simulink model "Assignment_2_simulink"  (R2025a)
settings: Solver=FixedStepDiscrete  StartTime=0.0  StopTime=inf  FixedStep=0.1  RelTol=1e-3  EnableMultiTasking=on
values from neighbouring files (symbols this model uses):
  Kv = 0.35    [Assignment_2.m]
  Kw = 2    [Assignment_2.m]
  Quaternion_Matrix = [waypoints(:, 1:2) Quaternion_Matrix]    [Assignment_2.m]
  tol = 0.05    [Assignment_2.m]
undefined symbols (not defined in the file or in its folder): twist
libraries: ros2lib x4
settings Model: Creator=arrigon88_msi_u24  LastModifiedBy=diego
settings OptimizationCC: DefaultParameterBehavior=Inlined  EnhancedBackFolding=on  PassReuseOutputArgsAs=Individual arguments  ZeroExternalMemoryAtStartup=off  ZeroInternalMemoryAtStartup=off  MaxStackSize=64  OptimizeBlockOrder=speed  DifferentSizesBufferReuse=on  OptimizationCustomize=off  EfficientTunableParamExpr=on
settings DebuggingCC: ParameterTunabilityLossMsg=error
settings HardwareCC: ProdBitPerLong=64.0  ProdHWDeviceType=Intel->x86-64 (Linux 64)
settings SFSimCC: MATLABDynamicMemAlloc=off
settings RTWCC: SystemTargetFile=ert.tlc  HardwareBoard=Robot Operating System 2 (ROS 2)  TLCOptions="-aInlineSetEventsForThisBaseRateFcn=TLC_FALSE -aSuppressMultiTaskScheduler=TLC_FALSE  -aRateBasedStepFcn=0"  TemplateMakefile=ert_default_tmf  Toolchain=Colcon Tools  TargetLang=C++  Description=Embedded Coder
settings CodeAppCC: ForceParamTrailComments=on  IgnoreCustomStorageClasses=off  OperatorAnnotations=on  SimulinkDataObjDesc=on  SFDataObjDesc=on  InsertBlockDesc=on
settings ERTTargetCC: ExtModeTransport=2.0  ExtModeAutomaticAllocSize=off  RootIOFormat=Structure reference  CodeInterfacePackaging=C++ class

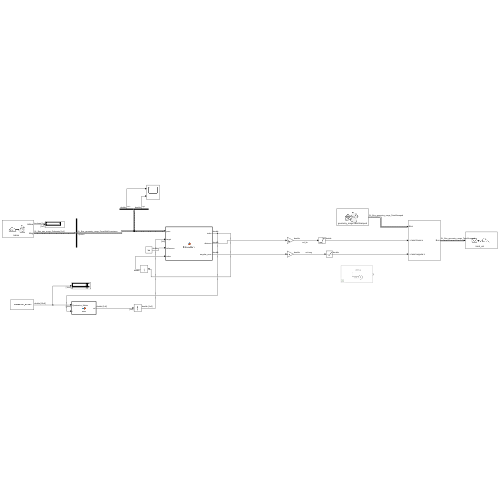
[thumbnail: Simulink's stored preview of the top-level diagram]
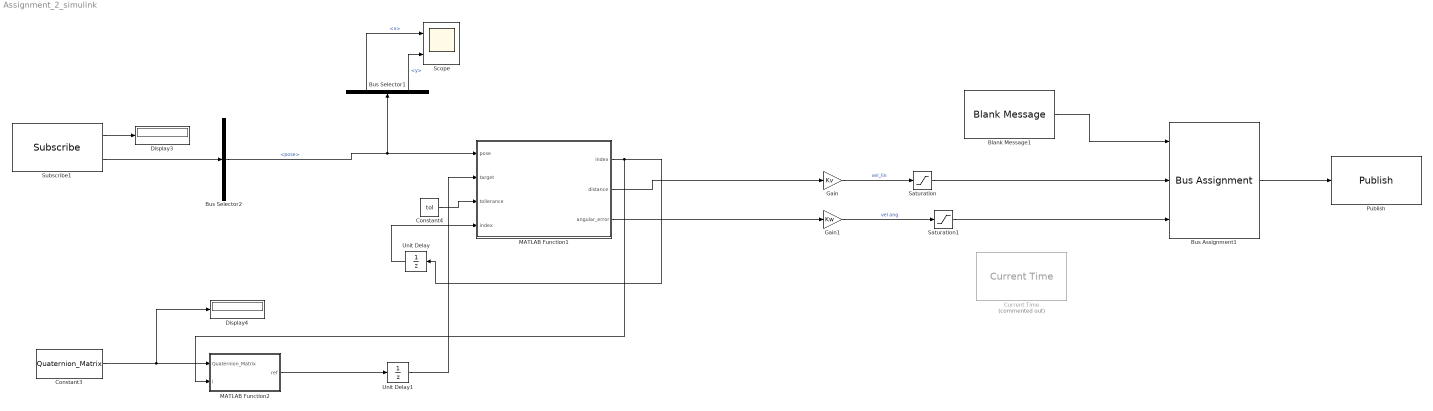
== system Assignment_2_simulink ==
  Blank Message1 : ros2lib/Blank Message  messageClass=Message  entityType=geometry_msgs/TwistStamped  messageType=geometry_msgs/TwistStamped  SampleTime=inf
  Bus Assignment1 : BusAssignment  AssignedSignals=twist.linear.x,twist.angular.z
  Bus Selector1 : BusSelector  OutputSignals=pose.position.x,pose.position.y
  Bus Selector2 : BusSelector  OutputSignals=pose
  Constant3 : Constant  Value=Quaternion_Matrix
  Constant4 : Constant  Value=tol
  Current Time : ros2lib/Current Time  Commented=on  OutputFormat=double  SampleTime=-1  ModelName=Assignment_2_simulink
  Display3 : Display
  Display4 : Display
  Gain : Gain  Gain=Kv
  Gain1 : Gain  Gain=Kw
  MATLAB Function1 : MATLAB Function  TreatAsAtomicUnit=on
  MATLAB Function2 : MATLAB Function  TreatAsAtomicUnit=on
  Publish : ros2lib/Publish  topicSource=Select from ROS network  topic=/cmd_vel  messageType=geometry_msgs/TwistStamped  QOSHistory=Keep last  QOSDepth=10  QOSReliability=Reliable  QOSDurability=Volatile  QOSDeadline=Inf  QOSLifespan=Inf  QOSLiveliness=Automatic  QOSLeaseDuration=Inf  QOSAvoidROSNamespaceConventions=off
  Saturation : Saturate  UpperLimit=0.2  LowerLimit=0
  Saturation1 : Saturate  UpperLimit=0.4  LowerLimit=0
  Scope : Scope  NumInputPorts=2
      settings: ActiveDisplayYMinimum=-1  ActiveDisplayYMaximum=1
  Subscribe1 : ros2lib/Subscribe  topicSource=Select from ROS network  topic=/odom  messageType=nav_msgs/Odometry  sampleTime=-1  QOSHistory=Keep last  QOSDepth=10  QOSReliability=Reliable  QOSDurability=Volatile  QOSDeadline=Inf  QOSLifespan=Inf  QOSLiveliness=Automatic  QOSLeaseDuration=Inf  QOSAvoidROSNamespaceConventions=off
  Unit Delay : UnitDelay  SampleTime=-1  HasFrameUpgradeWarning=on
  Unit Delay1 : UnitDelay  SampleTime=-1  HasFrameUpgradeWarning=on
  wires:
  Constant3/1 -> Display4/1, MATLAB Function2/1(Quaternion_Matrix)
  MATLAB Function1/1(index) -> Unit Delay/1, MATLAB Function2/2(i)
  Subscribe1/2 -> Bus Selector2/1
  Subscribe1/1 -> Display3/1
  MATLAB Function2/1(ref) -> Unit Delay1/1
  Constant4/1 -> MATLAB Function1/3(tollerance)
  MATLAB Function1/2(distance) -> Gain/1
  Gain/1 -> Saturation/1  "vel_lin"
  MATLAB Function1/3(angular_error) -> Gain1/1
  Gain1/1 -> Saturation1/1  "vel ang"
  Saturation/1 -> Bus Assignment1/2
  Blank Message1/1 -> Bus Assignment1/1
  Bus Assignment1/1 -> Publish/1
  Saturation1/1 -> Bus Assignment1/3
  Bus Selector2/1 -> Bus Selector1/1, MATLAB Function1/1(pose)  "<pose>"
  Unit Delay/1 -> MATLAB Function1/4("index ")
  Unit Delay1/1 -> MATLAB Function1/2(target)
  Bus Selector1/2 -> Scope/2  "<y>"
  Bus Selector1/1 -> Scope/1  "<x>"

== matlab function Assignment_2_simulink/MATLAB Function1 ==
  data: pose input; index output; target input; tollerance input; index input; distance output; angular_error output
function [index , distance , angular_error ]  = Interruttore(pose, target,tollerance, index)

% --- 2. Calcolo Distanza (Corretto) ---
    % Estrai X,Y da 'position' (Bus/Struct)
    pos_attuale = [pose.pose.position.x, pose.pose.position.y];
    angular_error = 0;
    % Estrai X,Y da 'target' (Array)
    pos_target = [target(1), target(2)];
    
    % Calcola la distanza 2D
    distance = norm(pos_attuale - pos_target);

    if distance<tollerance
       distance = 0;
     angular_error =  norm(target(3:6) - pose.pose.orientation.z) ;
     if angular_error<0.005
       index = index + 1;
       angular_error = 0;
     end
    end
end

== matlab function Assignment_2_simulink/MATLAB Function2 ==
  data: Quaternion_Matrix input; i input; ref output
function ref = fcn( Quaternion_Matrix, i)

ref = Quaternion_Matrix(i,:);
